simulink model "Sementation_4K_480p"  (R2021a)
settings: Solver=FixedStepDiscrete  StartTime=0.0  StopTime=1000  RelTol=1e-3
InitFcn:
  | Ts = 1e-3;
  | Ts_240p = 402*324*Ts;
  | Ts_480p = 525*800*Ts;
undefined symbols (not defined in the file or in its folder): gray, Rec, SDTV
libraries: hdlsllib x10, visionhdlio x2, visionhdlconversions x2, dspvision x1
settings Model: DataTypeOverride=Off  ModifiedByFormat=The MathWorks Inc.  NumberOfSteps=10  Creator=The MathWorks, Inc.  LastModifiedBy=The MathWorks Inc.
settings SolverCC: AlgebraicLoopSolver=TrustRegion
settings DataIOCC: LimitDataPoints=on  SaveFormat=Array  SaveOutput=off  SaveTime=off  ReturnWorkspaceOutputs=off
settings OptimizationCC: BlockReduction=off  ConditionallyExecuteInputs=off  DefaultParameterBehavior=Inlined  LifeSpan=inf
settings DebuggingCC: AlgebraicLoopMsg=error  SolverPrmCheckMsg=warning  SingleTaskRateTransMsg=error  ParameterPrecisionLossMsg=none  AllowSymbolicDim=off  SFUnexpectedBacktrackingDiag=warning  SFNoUnconditionalDefaultTransitionDiag=warning  SFExecutionAtInitializationDiag=none  SFMachineParentedDataDiag=warning  IntegerSaturationMsg=none  ArithmeticOperatorsInVariantConditions=warning
settings HardwareCC: ProdBitPerPointer=32  ProdBitPerSizeT=32  ProdBitPerPtrDiffT=32  ProdLargestAtomicFloat=None  ProdIntDivRoundTo=Undefined  ProdEndianess=Unspecified  ProdWordSize=32  ProdHWDeviceType=ASIC/FPGA->ASIC/FPGA  ProdEqTarget=off
settings ModelReferenceCC: PropagateSignalLabelsOutOfModel=off
settings SFSimCC: SimUseLocalCustomCode=off  CustomCodeUndefinedFunction=UseInterfaceOnly
settings RTWCC: RTWUseLocalCustomCode=off
settings CodeAppCC: StateflowObjectComments=on
settings GRTTargetCC: TargetLangStandard=C89/C90 (ANSI)
settings ConfigComp: CovMetricSettings=dw  CovSaveCumulativeToWorkspaceVar=on  CovSaveSingleToWorkspaceVar=on  CovExternalEMLEnable=off  CovSFcnEnable=off

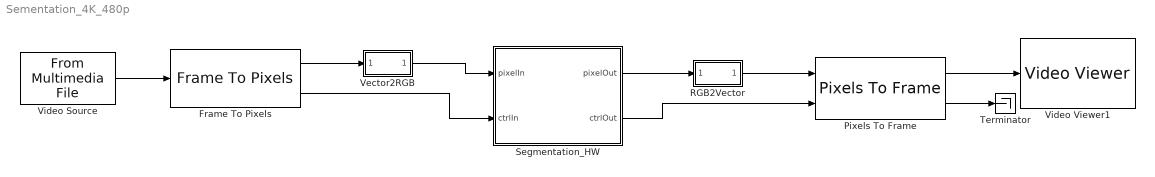
== system Sementation_4K_480p ==
  Frame To Pixels : visionhdlio/Frame To Pixels  NumComponents=3  NumPixels=1  VideoFormat=480p  ActivePixelsPerLine=32  ActiveVideoLines=18  TotalPixelsPerLine=42  TotalVideoLines=28  StartingActiveLine=6  FrontPorch=5  SampleTime=0
      settings: SourceProductBaseCode=VT
  Pixels To Frame : visionhdlio/Pixels To Frame  NumComponents=3  NumPixels=1  VideoFormat=480p  ActivePixelsPerLine=32  ActiveVideoLines=18  TotalPixelsPerLine=42  TotalVideoLines=28
      settings: SourceProductBaseCode=VT
  RGB2Vector : Subsystem
  Segmentation_HW : Subsystem  TreatAsAtomicUnit=on
  Terminator : Terminator
  Vector2RGB : Subsystem
  Video Source : dspvision/From Multimedia File  inputFilename=D:\Work\XilFPGAdev\Custom_IP_Cores\SimulinkHDLCoder\testImages\mountain_480p.jpg  readRange=[1 Inf]  loop=on  numPlays=inf  outputStreams=Video only  videoDataType=uint8  audioDataType=int16  inheritSampleTime=off  userDefinedSampleTime=0.001  noAudioOutput=off  isIntensityVideo=off  fourcc=RGB  colorVideoFormat=One multidimensional signal  outputEOF=off  dataOrg=Column-major  audioFrameSize=1024  computeAudioFrameSize=off  outSamplingMode=Sample based
  Video Viewer1 : VideoViewer  colormapValue=gray(256)  FigPos=[838 665 498 402]
  wires:
  Pixels To Frame/2 -> Terminator/1
  Pixels To Frame/1 -> Video Viewer1/1
  Vector2RGB/1(RGB) -> Segmentation_HW/1(pixelIn)
  Segmentation_HW/1(pixelOut) -> RGB2Vector/1(RGB)
  Video Source/1 -> Frame To Pixels/1
  Frame To Pixels/2 -> Segmentation_HW/2(ctrlIn)
  Frame To Pixels/1 -> Vector2RGB/1(RGBVector)
  RGB2Vector/1(RGBVector) -> Pixels To Frame/1
  Segmentation_HW/2(ctrlOut) -> Pixels To Frame/2

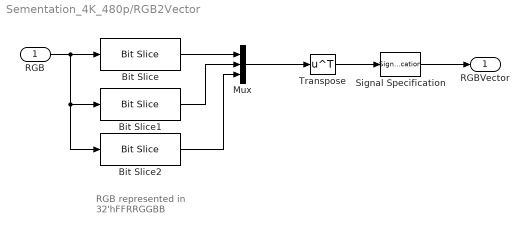
== system Sementation_4K_480p/RGB2Vector ==
  note: RGB represented in
      | 32'hFFRRGGBB
  RGB : Inport
  Bit Slice : hdlsllib/Logic and Bit Operations/Bit Slice  lidx=23  ridx=16
      settings: SourceProductBaseCode=SL
  Bit Slice1 : hdlsllib/Logic and Bit Operations/Bit Slice  lidx=15  ridx=8
      settings: SourceProductBaseCode=SL
  Bit Slice2 : hdlsllib/Logic and Bit Operations/Bit Slice  lidx=7  ridx=0
      settings: SourceProductBaseCode=SL
  Mux : Mux  Inputs=3
  Signal Specification : SignalSpecification
  Transpose : Math  Operator=transpose  SignedPower=on  SaturateOnIntegerOverflow=on
  RGBVector : Outport  VectorParamsAs1DForOutWhenUnconnected=off
  wires:
  Mux/1 -> Transpose/1
  Bit Slice/1 -> Mux/1
  Bit Slice2/1 -> Mux/3
  Bit Slice1/1 -> Mux/2
  RGB/1 -> Bit Slice2/1, Bit Slice1/1, Bit Slice/1
  Transpose/1 -> Signal Specification/1
  Signal Specification/1 -> RGBVector/1

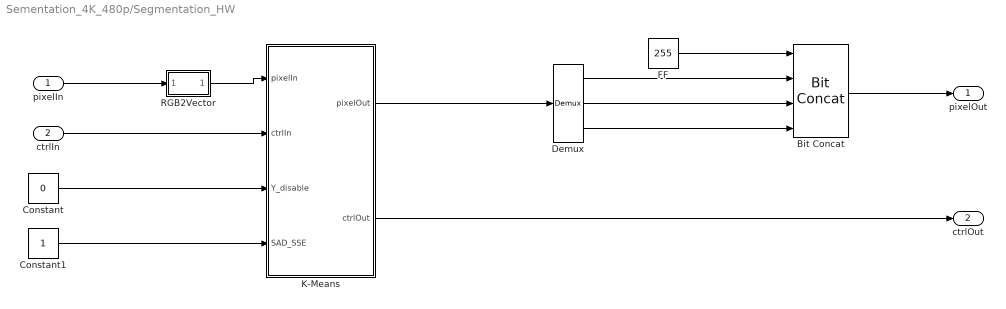
== system Sementation_4K_480p/Segmentation_HW ==
  pixelIn : Inport
  ctrlIn : Inport  Port=2
  Bit Concat : hdlsllib/Logic and Bit Operations/Bit Concat  numInputs=4
  Constant : Constant  Value=0  OutDataTypeStr=uint8
  Constant1 : Constant  OutDataTypeStr=uint8
  Demux : Demux  Outputs=3
  FF : Constant  Value=255  OutDataTypeStr=uint8  SampleTime=-1
  K-Means : Subsystem  TreatAsAtomicUnit=on
  RGB2Vector : Subsystem
  pixelOut : Outport  VectorParamsAs1DForOutWhenUnconnected=off
  ctrlOut : Outport  Port=2  VectorParamsAs1DForOutWhenUnconnected=off
  wires:
  ctrlIn/1 -> K-Means/2(ctrlIn)
  pixelIn/1 -> RGB2Vector/1(RGB)
  RGB2Vector/1(RGBVector) -> K-Means/1(pixelIn)
  FF/1 -> Bit Concat/1
  Bit Concat/1 -> pixelOut/1
  Demux/3 -> Bit Concat/4
  Demux/2 -> Bit Concat/3
  Demux/1 -> Bit Concat/2
  K-Means/2(ctrlOut) -> ctrlOut/1
  K-Means/1(pixelOut) -> Demux/1
  Constant/1 -> K-Means/3(Y_disable)
  Constant1/1 -> K-Means/4(SAD_SSE)

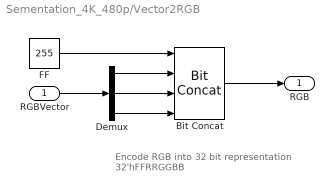
== system Sementation_4K_480p/Vector2RGB ==
  note: Encode RGB into 32 bit representation
      | 32'hFFRRGGBB
  RGBVector : Inport
  Bit Concat : hdlsllib/Logic and Bit Operations/Bit Concat  numInputs=4
  Demux : Demux  Outputs=3
  FF : Constant  Value=255  OutDataTypeStr=uint8  SampleTime=-1
  RGB : Outport  VectorParamsAs1DForOutWhenUnconnected=off
  wires:
  Bit Concat/1 -> RGB/1
  RGBVector/1 -> Demux/1
  FF/1 -> Bit Concat/1
  Demux/1 -> Bit Concat/2
  Demux/2 -> Bit Concat/3
  Demux/3 -> Bit Concat/4

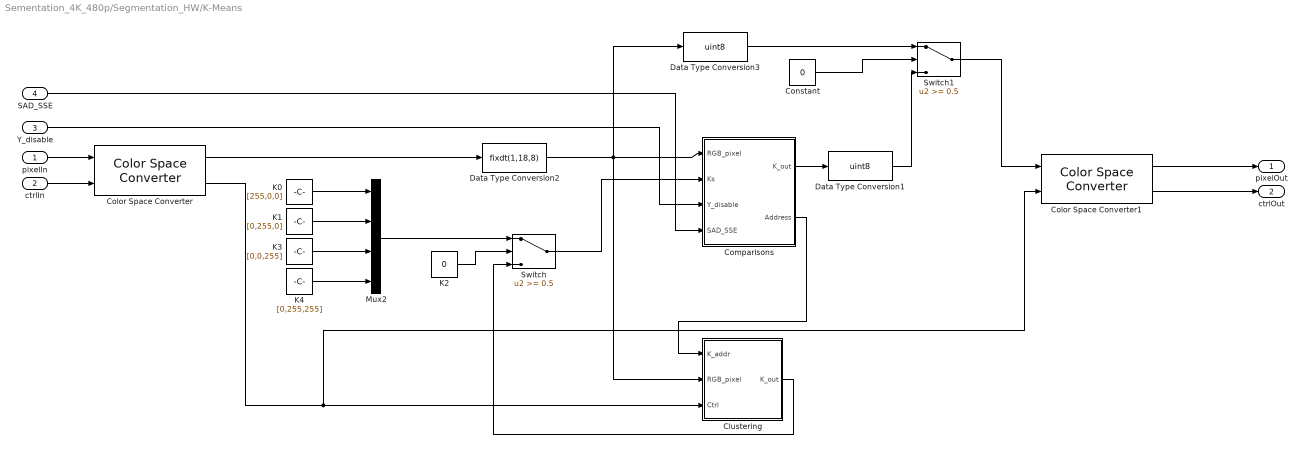
== system Sementation_4K_480p/Segmentation_HW/K-Means ==
  pixelIn : Inport
  ctrlIn : Inport  Port=2
  Y_disable : Inport  Port=3
  SAD_SSE : Inport  Port=4
  Clustering : Subsystem
  Color Space Converter : visionhdlconversions/Color Space Converter  Conversion=RGB to YCbCr  ConversionStandard=Rec. 601 (SDTV)  ScanningStandard=1250/50/2:1  SimulateUsing=Code generation
      settings: SourceProductBaseCode=VT
  Color Space Converter1 : visionhdlconversions/Color Space Converter  Conversion=YCbCr to RGB  ConversionStandard=Rec. 601 (SDTV)  ScanningStandard=1250/50/2:1  SimulateUsing=Code generation
      settings: SourceProductBaseCode=VT
  Comparisons : Subsystem
  Constant : Constant  Value=0  OutDataTypeStr=uint8
  Data Type Conversion1 : DataTypeConversion  OutDataTypeStr=uint8  RndMeth=Nearest
  Data Type Conversion2 : DataTypeConversion  OutDataTypeStr=fixdt(1,18,8)  RndMeth=Nearest
  Data Type Conversion3 : DataTypeConversion  OutDataTypeStr=uint8  RndMeth=Nearest
  K0 : Constant  Value=[255,0,0]  OutDataTypeStr=fixdt(1,18,8)
  K1 : Constant  Value=[0,255,0]  OutDataTypeStr=fixdt(1,18,8)
  K2 : Constant  Value=0  OutDataTypeStr=uint8
  K3 : Constant  Value=[0,0,255]  OutDataTypeStr=fixdt(1,18,8)
  K4 : Constant  Value=[0,255,255]  OutDataTypeStr=fixdt(1,18,8)
  Mux2 : Mux
  Switch : Switch  Threshold=0.5
  Switch1 : Switch  Threshold=0.5
  pixelOut : Outport  VectorParamsAs1DForOutWhenUnconnected=off
  ctrlOut : Outport  Port=2  VectorParamsAs1DForOutWhenUnconnected=off
  wires:
  K2/1 -> Switch/2
  K0/1 -> Mux2/1
  K1/1 -> Mux2/2
  Mux2/1 -> Switch/1
  Switch/1 -> Comparisons/2(Ks)
  K3/1 -> Mux2/3
  K4/1 -> Mux2/4
  Comparisons/2(Address) -> Clustering/1(K_addr)
  Clustering/1(K_out) -> Switch/3
  pixelIn/1 -> Color Space Converter/1
  ctrlIn/1 -> Color Space Converter/2
  Color Space Converter/2 -> Color Space Converter1/2, Clustering/3(Ctrl)
  Color Space Converter1/1 -> pixelOut/1
  Color Space Converter1/2 -> ctrlOut/1
  Comparisons/1(K_out) -> Data Type Conversion1/1
  Switch1/1 -> Color Space Converter1/1
  Constant/1 -> Switch1/2
  Color Space Converter/1 -> Data Type Conversion2/1
  Data Type Conversion3/1 -> Switch1/1
  Data Type Conversion1/1 -> Switch1/3
  Y_disable/1 -> Comparisons/3(Y_disable)
  Data Type Conversion2/1 -> Data Type Conversion3/1, Clustering/2(RGB_pixel), Comparisons/1(RGB_pixel)
  SAD_SSE/1 -> Comparisons/4(SAD_SSE)

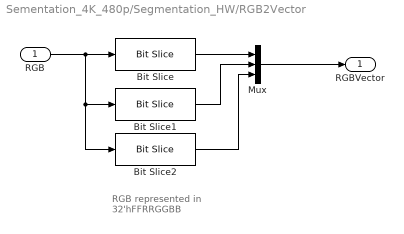
== system Sementation_4K_480p/Segmentation_HW/RGB2Vector ==
  note: RGB represented in
      | 32'hFFRRGGBB
  RGB : Inport
  Bit Slice : hdlsllib/Logic and Bit Operations/Bit Slice  lidx=23  ridx=16
      settings: SourceProductBaseCode=SL
  Bit Slice1 : hdlsllib/Logic and Bit Operations/Bit Slice  lidx=15  ridx=8
      settings: SourceProductBaseCode=SL
  Bit Slice2 : hdlsllib/Logic and Bit Operations/Bit Slice  lidx=7  ridx=0
      settings: SourceProductBaseCode=SL
  Mux : Mux  Inputs=3
  RGBVector : Outport  VectorParamsAs1DForOutWhenUnconnected=off
  wires:
  Bit Slice/1 -> Mux/1
  Bit Slice2/1 -> Mux/3
  Bit Slice1/1 -> Mux/2
  RGB/1 -> Bit Slice2/1, Bit Slice1/1, Bit Slice/1
  Mux/1 -> RGBVector/1

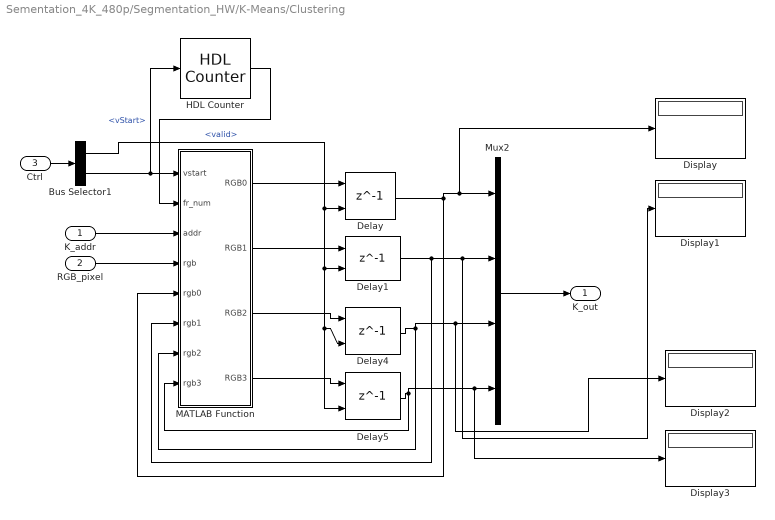
== system Sementation_4K_480p/Segmentation_HW/K-Means/Clustering ==
  K_addr : Inport
  RGB_pixel : Inport  Port=2
  Ctrl : Inport  Port=3
  Bus Selector1 : BusSelector  OutputSignals=valid,vStart
  Delay{,1,4..5} (4 alike) : Delay  DelayLength=1  InitialCondition=0  ShowEnablePort=on
      settings: InputPortMap=u0,e6
  Display{,1..3} (4 alike) : Display
  HDL Counter : hdlsllib/Sources/HDL Counter  CountType=Free running  CountInit=0  CountStep=1  CountMax=4  CountFromType=Initial value  CountFrom=0  CountResetPort=off  CountLoadPort=off  CountEnbPort=on  CountDirPort=off  CountHitOutputPort=off  CountDataType=Unsigned  CountWordLen=12  CountFracLen=0  CountSampTime=1
  MATLAB Function : MATLAB Function  TreatAsAtomicUnit=on
  Mux2 : Mux
  K_out : Outport  VectorParamsAs1DForOutWhenUnconnected=off
  wires:
  Delay5/1 -> Display3/1, Mux2/4, MATLAB Function/8(rgb3)
  K_addr/1 -> MATLAB Function/3(addr)
  Bus Selector1/1 -> Delay5/2, Delay4/2, Delay1/2, Delay/2  "<valid>"
  MATLAB Function/2(RGB1) -> Delay1/1
  Delay4/1 -> Display2/1, Mux2/3, MATLAB Function/7(rgb2)
  Bus Selector1/2 -> HDL Counter/1, MATLAB Function/1(vstart)  "<vStart>"
  MATLAB Function/1(RGB0) -> Delay/1
  Delay1/1 -> MATLAB Function/6(rgb1), Display1/1, Mux2/2
  Delay/1 -> Display/1, Mux2/1, MATLAB Function/5(rgb0)
  RGB_pixel/1 -> MATLAB Function/4(rgb)
  Ctrl/1 -> Bus Selector1/1
  MATLAB Function/3(RGB2) -> Delay4/1
  MATLAB Function/4(RGB3) -> Delay5/1
  HDL Counter/1 -> MATLAB Function/2(fr_num)
  Mux2/1 -> K_out/1

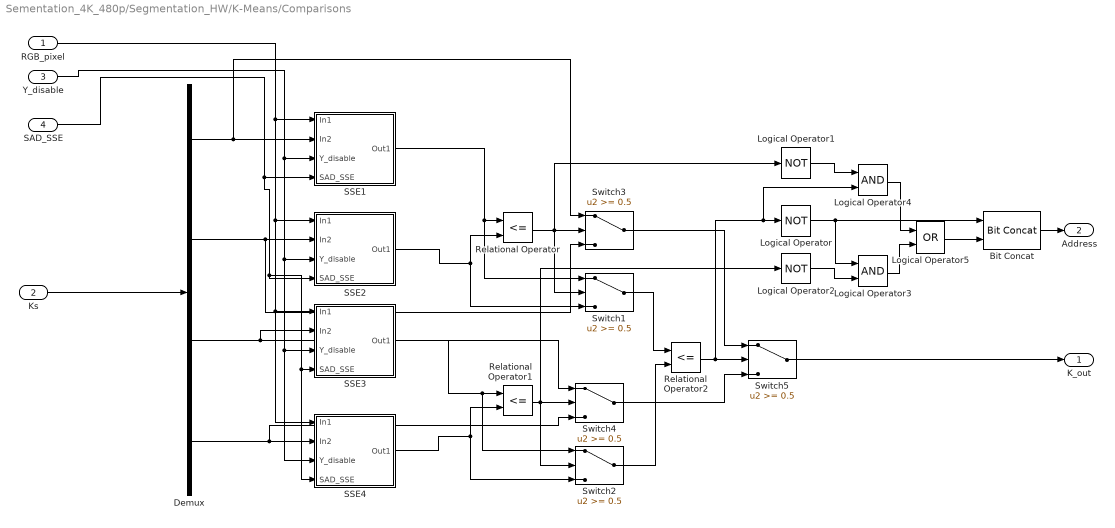
== system Sementation_4K_480p/Segmentation_HW/K-Means/Comparisons ==
  RGB_pixel : Inport
  Ks : Inport  Port=2
  Y_disable : Inport  Port=3
  SAD_SSE : Inport  Port=4
  Bit Concat : hdlsllib/Logic and Bit Operations/Bit Concat  numInputs=2
  Demux : Demux
  Logical Operator : Logic  Operator=NOT  AllPortsSameDT=off  OutDataTypeStr=boolean
  Logical Operator1 : Logic  Operator=NOT  AllPortsSameDT=off  OutDataTypeStr=boolean
  Logical Operator2 : Logic  Operator=NOT  AllPortsSameDT=off  OutDataTypeStr=boolean
  Logical Operator3 : Logic  AllPortsSameDT=off  OutDataTypeStr=boolean
  Logical Operator4 : Logic  AllPortsSameDT=off  OutDataTypeStr=boolean
  Logical Operator5 : Logic  Operator=OR  AllPortsSameDT=off  OutDataTypeStr=boolean
  Relational Operator : RelationalOperator  Operator=<=  OutDataTypeStr=boolean  RndMeth=Nearest
  Relational Operator1 : RelationalOperator  Operator=<=  OutDataTypeStr=boolean  RndMeth=Nearest
  Relational Operator2 : RelationalOperator  Operator=<=  OutDataTypeStr=boolean  RndMeth=Nearest
  SSE1 : Subsystem
  SSE2 : Subsystem
  SSE3 : Subsystem
  SSE4 : Subsystem
  Switch{1..5} (5 alike) : Switch  Threshold=0.5
  K_out : Outport  VectorParamsAs1DForOutWhenUnconnected=off
  Address : Outport  Port=2  VectorParamsAs1DForOutWhenUnconnected=off
  wires:
  Ks/1 -> Demux/1
  RGB_pixel/1 -> SSE1/1(In1), SSE2/1(In1), SSE3/1(In1), SSE4/1(In1)
  Demux/1 -> Switch3/1, SSE1/2(In2)
  Demux/2 -> SSE2/2(In2), Switch3/3
  Demux/3 -> SSE3/2(In2), Switch4/1
  Demux/4 -> Switch4/3, SSE4/2(In2)
  SSE1/1(Out1) -> Switch1/1, Relational Operator/1
  SSE2/1(Out1) -> Switch1/3, Relational Operator/2
  SSE4/1(Out1) -> Switch2/3, Relational Operator1/2
  Relational Operator/1 -> Logical Operator1/1, Switch1/2, Switch3/2
  Relational Operator1/1 -> Logical Operator2/1, Switch2/2, Switch4/2
  Switch5/1 -> K_out/1
  SSE3/1(Out1) -> Switch2/1, Relational Operator1/1
  Relational Operator2/1 -> Switch5/2, Logical Operator4/2, Logical Operator/1
  Switch1/1 -> Relational Operator2/1
  Switch2/1 -> Relational Operator2/2
  Switch3/1 -> Switch5/1
  Switch4/1 -> Switch5/3
  Logical Operator/1 -> Logical Operator3/1, Bit Concat/1
  Logical Operator2/1 -> Logical Operator3/2
  Logical Operator1/1 -> Logical Operator4/1
  Logical Operator3/1 -> Logical Operator5/2
  Logical Operator4/1 -> Logical Operator5/1
  Logical Operator5/1 -> Bit Concat/2
  Bit Concat/1 -> Address/1
  Y_disable/1 -> SSE1/3(Y_disable), SSE2/3(Y_disable), SSE4/3(Y_disable), SSE3/3(Y_disable)
  SAD_SSE/1 -> SSE4/4(SAD_SSE), SSE3/4(SAD_SSE), SSE2/4(SAD_SSE), SSE1/4(SAD_SSE)

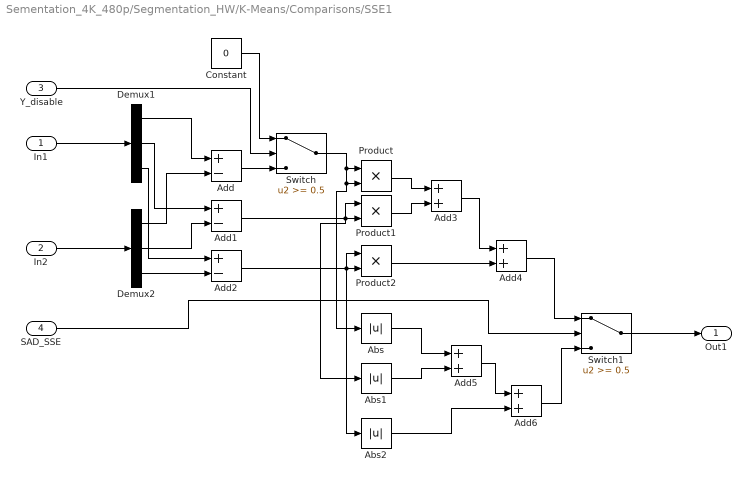
== system Sementation_4K_480p/Segmentation_HW/K-Means/Comparisons/SSE1 ==
  In1 : Inport
  In2 : Inport  Port=2
  Y_disable : Inport  Port=3
  SAD_SSE : Inport  Port=4
  Abs : Abs
  Abs1 : Abs
  Abs2 : Abs
  Add : Sum  Inputs=+-  OutDataTypeStr=Inherit: Inherit via back propagation
  Add1 : Sum  Inputs=+-  OutDataTypeStr=Inherit: Inherit via back propagation
  Add2 : Sum  Inputs=+-  OutDataTypeStr=Inherit: Inherit via back propagation
  Add{3..6} (4 alike) : Sum
  Constant : Constant  Value=0  OutDataTypeStr=fixdt(1,18,8)
  Demux1 : Demux  Outputs=3
  Demux2 : Demux  Outputs=3
  Product : Product
  Product1 : Product
  Product2 : Product
  Switch : Switch  Threshold=0.5
  Switch1 : Switch  Threshold=0.5
  Out1 : Outport  VectorParamsAs1DForOutWhenUnconnected=off
  wires:
  Product/1 -> Add3/1
  Demux2/2 -> Add1/2
  Product2/1 -> Add4/2
  Product1/1 -> Add3/2
  Add3/1 -> Add4/1
  Demux2/1 -> Add/2
  Demux1/3 -> Add2/1
  Add1/1 -> Abs1/1, Product1/2, Product1/1
  Add2/1 -> Abs2/1, Product2/2, Product2/1
  Demux2/3 -> Add2/2
  Demux1/2 -> Add1/1
  Demux1/1 -> Add/1
  In1/1 -> Demux1/1
  In2/1 -> Demux2/1
  Constant/1 -> Switch/1
  Add/1 -> Switch/3
  Switch/1 -> Abs/1, Product/2, Product/1
  Y_disable/1 -> Switch/2
  Add4/1 -> Switch1/1
  SAD_SSE/1 -> Switch1/2
  Abs/1 -> Add5/1
  Abs1/1 -> Add5/2
  Add5/1 -> Add6/1
  Abs2/1 -> Add6/2
  Switch1/1 -> Out1/1
  Add6/1 -> Switch1/3

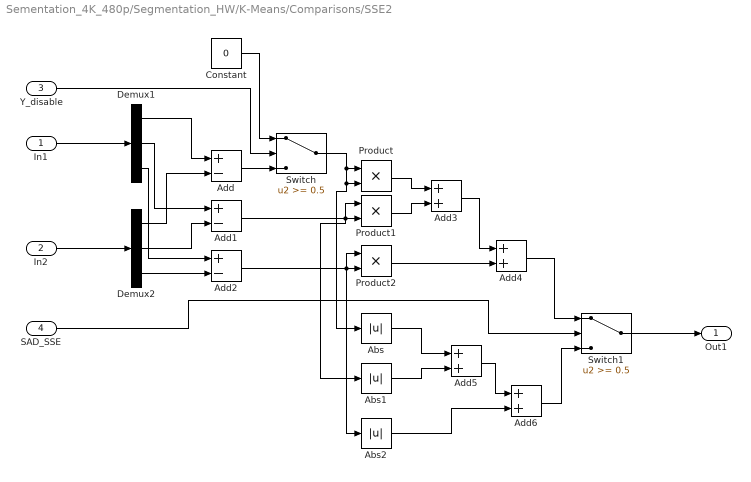
== system Sementation_4K_480p/Segmentation_HW/K-Means/Comparisons/SSE2 ==
  In1 : Inport
  In2 : Inport  Port=2
  Y_disable : Inport  Port=3
  SAD_SSE : Inport  Port=4
  Abs : Abs
  Abs1 : Abs
  Abs2 : Abs
  Add : Sum  Inputs=+-  OutDataTypeStr=Inherit: Inherit via back propagation
  Add1 : Sum  Inputs=+-  OutDataTypeStr=Inherit: Inherit via back propagation
  Add2 : Sum  Inputs=+-  OutDataTypeStr=Inherit: Inherit via back propagation
  Add{3..6} (4 alike) : Sum
  Constant : Constant  Value=0  OutDataTypeStr=fixdt(1,18,8)
  Demux1 : Demux  Outputs=3
  Demux2 : Demux  Outputs=3
  Product : Product
  Product1 : Product
  Product2 : Product
  Switch : Switch  Threshold=0.5
  Switch1 : Switch  Threshold=0.5
  Out1 : Outport  VectorParamsAs1DForOutWhenUnconnected=off
  wires:
  Product/1 -> Add3/1
  Demux2/2 -> Add1/2
  Product2/1 -> Add4/2
  Product1/1 -> Add3/2
  Add3/1 -> Add4/1
  Demux2/1 -> Add/2
  Demux1/3 -> Add2/1
  Add1/1 -> Abs1/1, Product1/2, Product1/1
  Add2/1 -> Abs2/1, Product2/2, Product2/1
  Demux2/3 -> Add2/2
  Demux1/2 -> Add1/1
  Demux1/1 -> Add/1
  In1/1 -> Demux1/1
  In2/1 -> Demux2/1
  Constant/1 -> Switch/1
  Add/1 -> Switch/3
  Switch/1 -> Abs/1, Product/2, Product/1
  Y_disable/1 -> Switch/2
  Add4/1 -> Switch1/1
  SAD_SSE/1 -> Switch1/2
  Abs/1 -> Add5/1
  Abs1/1 -> Add5/2
  Add5/1 -> Add6/1
  Abs2/1 -> Add6/2
  Switch1/1 -> Out1/1
  Add6/1 -> Switch1/3

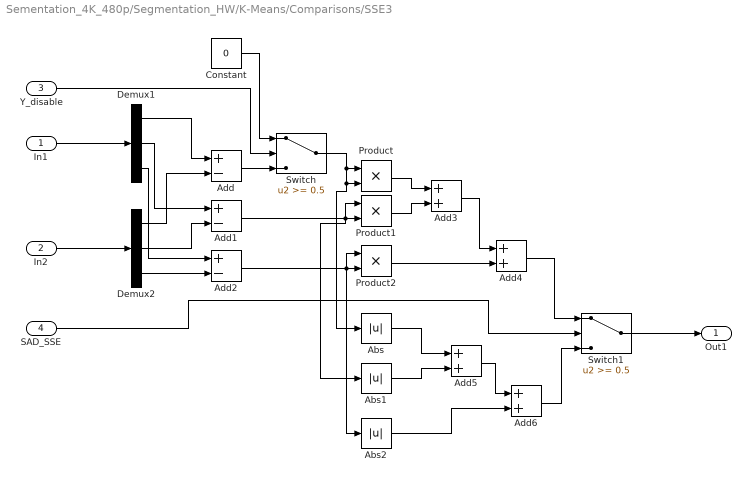
== system Sementation_4K_480p/Segmentation_HW/K-Means/Comparisons/SSE3 ==
  In1 : Inport
  In2 : Inport  Port=2
  Y_disable : Inport  Port=3
  SAD_SSE : Inport  Port=4
  Abs : Abs
  Abs1 : Abs
  Abs2 : Abs
  Add : Sum  Inputs=+-  OutDataTypeStr=Inherit: Inherit via back propagation
  Add1 : Sum  Inputs=+-  OutDataTypeStr=Inherit: Inherit via back propagation
  Add2 : Sum  Inputs=+-  OutDataTypeStr=Inherit: Inherit via back propagation
  Add{3..6} (4 alike) : Sum
  Constant : Constant  Value=0  OutDataTypeStr=fixdt(1,18,8)
  Demux1 : Demux  Outputs=3
  Demux2 : Demux  Outputs=3
  Product : Product
  Product1 : Product
  Product2 : Product
  Switch : Switch  Threshold=0.5
  Switch1 : Switch  Threshold=0.5
  Out1 : Outport  VectorParamsAs1DForOutWhenUnconnected=off
  wires:
  Product/1 -> Add3/1
  Demux2/2 -> Add1/2
  Product2/1 -> Add4/2
  Product1/1 -> Add3/2
  Add3/1 -> Add4/1
  Demux2/1 -> Add/2
  Demux1/3 -> Add2/1
  Add1/1 -> Abs1/1, Product1/2, Product1/1
  Add2/1 -> Abs2/1, Product2/2, Product2/1
  Demux2/3 -> Add2/2
  Demux1/2 -> Add1/1
  Demux1/1 -> Add/1
  In1/1 -> Demux1/1
  In2/1 -> Demux2/1
  Constant/1 -> Switch/1
  Add/1 -> Switch/3
  Switch/1 -> Abs/1, Product/2, Product/1
  Y_disable/1 -> Switch/2
  Add4/1 -> Switch1/1
  SAD_SSE/1 -> Switch1/2
  Abs/1 -> Add5/1
  Abs1/1 -> Add5/2
  Add5/1 -> Add6/1
  Abs2/1 -> Add6/2
  Switch1/1 -> Out1/1
  Add6/1 -> Switch1/3

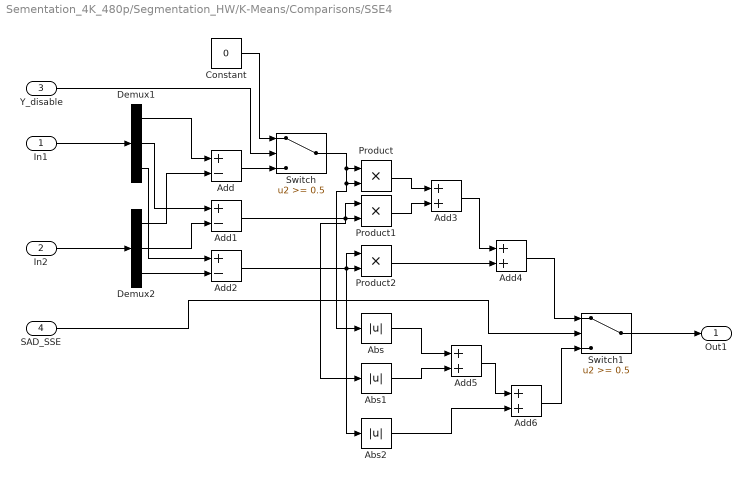
== system Sementation_4K_480p/Segmentation_HW/K-Means/Comparisons/SSE4 ==
  In1 : Inport
  In2 : Inport  Port=2
  Y_disable : Inport  Port=3
  SAD_SSE : Inport  Port=4
  Abs : Abs
  Abs1 : Abs
  Abs2 : Abs
  Add : Sum  Inputs=+-  OutDataTypeStr=Inherit: Inherit via back propagation
  Add1 : Sum  Inputs=+-  OutDataTypeStr=Inherit: Inherit via back propagation
  Add2 : Sum  Inputs=+-  OutDataTypeStr=Inherit: Inherit via back propagation
  Add{3..6} (4 alike) : Sum
  Constant : Constant  Value=0  OutDataTypeStr=fixdt(1,18,8)
  Demux1 : Demux  Outputs=3
  Demux2 : Demux  Outputs=3
  Product : Product
  Product1 : Product
  Product2 : Product
  Switch : Switch  Threshold=0.5
  Switch1 : Switch  Threshold=0.5
  Out1 : Outport  VectorParamsAs1DForOutWhenUnconnected=off
  wires:
  Product/1 -> Add3/1
  Demux2/2 -> Add1/2
  Product2/1 -> Add4/2
  Product1/1 -> Add3/2
  Add3/1 -> Add4/1
  Demux2/1 -> Add/2
  Demux1/3 -> Add2/1
  Add1/1 -> Abs1/1, Product1/2, Product1/1
  Add2/1 -> Abs2/1, Product2/2, Product2/1
  Demux2/3 -> Add2/2
  Demux1/2 -> Add1/1
  Demux1/1 -> Add/1
  In1/1 -> Demux1/1
  In2/1 -> Demux2/1
  Constant/1 -> Switch/1
  Add/1 -> Switch/3
  Switch/1 -> Abs/1, Product/2, Product/1
  Y_disable/1 -> Switch/2
  Add4/1 -> Switch1/1
  SAD_SSE/1 -> Switch1/2
  Abs/1 -> Add5/1
  Abs1/1 -> Add5/2
  Add5/1 -> Add6/1
  Abs2/1 -> Add6/2
  Switch1/1 -> Out1/1
  Add6/1 -> Switch1/3

== matlab function Sementation_4K_480p/Segmentation_HW/K-Means/Clustering/MATLAB Function ==
  data: vstart input; fr_num input; addr input; rgb input; RGB0 output fixdt(1,18,8) size=[1,3]; rgb0 input; rgb1 input; RGB1 output fixdt(1,18,8) size=[1,3]; rgb2 input; rgb3 input; RGB2 output fixdt(1,18,8) size=[1,3]; RGB3 output fixdt(1,18,8) size=[1,3]
function [RGB0,RGB1,RGB2,RGB3] = fcn(vstart,fr_num,addr,rgb,rgb0,rgb1,rgb2,rgb3)

alpha = fi(0.999);
rgb_alpha = (rgb)*fi(fi(1)-alpha);
rgb00 = fi(rgb0,1,18,8);
rgb11 = fi(rgb1,1,18,8);
rgb22 = fi(rgb2,1,18,8);
rgb33 = fi(rgb3,1,18,8);

if(vstart&(fr_num==0))
    RGB00 = fi([127,127,127],1,18,8);
    RGB11 = fi([127,127,127],1,18,8);
    RGB22 = fi([127,127,127],1,18,8);
    RGB33 = fi([127,127,127],1,18,8);
else
    if(addr==0)
        RGB00 = fi(rgb00*alpha + rgb_alpha,1,18,8);
        RGB11 = rgb11;
        RGB22 = rgb22;
        RGB33 = rgb33;
    elseif(addr==1)
        RGB00 = rgb00;
        RGB11 = fi(rgb11*alpha + rgb_alpha,1,18,8);
        RGB22 = rgb22;
        RGB33 = rgb33;
    elseif(addr==2)
        RGB00 = rgb00;
        RGB11 = rgb11;
        RGB22 = fi(rgb22*alpha + rgb_alpha,1,18,8);
        RGB33 = rgb33;
    else
        RGB00 = rgb00;
        RGB11 = rgb11;
        RGB22 = rgb22;
        RGB33 = fi(rgb33*alpha + rgb_alpha,1,18,8);
    end
end

RGB0 = fi(RGB00,1,18,8);
RGB1 = fi(RGB11,1,18,8);
RGB2 = fi(RGB22,1,18,8);
RGB3 = fi(RGB33,1,18,8);
